simulink model "P1sim"  (R2020b)
settings: Solver=VariableStepAuto  StartTime=0.0  StopTime=100  RelTol=1e-3
undefined symbols (not defined in the file): A, B, C, den, ftDisc, ftPIDdisc, kd1, Kesc, ki, ki2, kp, Kram, num, rampCER, rampPOL, wMuestr
settings Model: Creator=Julian  LastModifiedBy=Julian

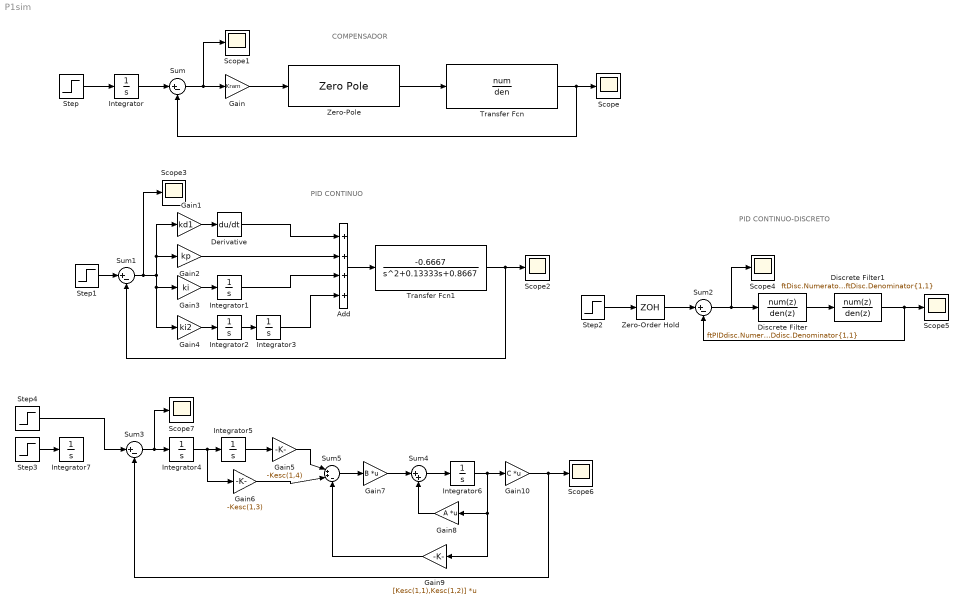
== system P1sim ==
  note: PID CONTINUO-DISCRETO
  note: PID CONTINUO
  note: COMPENSADOR
  Add : Sum  Inputs=++++
  Derivative : Derivative
  Discrete Filter : DiscreteFilter  Numerator=ftPIDdisc.Numerator{1,1}  Denominator=ftPIDdisc.Denominator{1,1}
  Discrete Filter1 : DiscreteFilter  Numerator=ftDisc.Numerator{1,1}  Denominator=ftDisc.Denominator{1,1}
  Gain : Gain  Gain=Kram
  Gain1 : Gain  Gain=kd1
  Gain10 : Gain  Gain=C  Multiplication=Matrix(K*u)
  Gain2 : Gain  Gain=kp
  Gain3 : Gain  Gain=ki
  Gain4 : Gain  Gain=ki2
  Gain5 : Gain  Gain=-Kesc(1,4)
  Gain6 : Gain  Gain=-Kesc(1,3)
  Gain7 : Gain  Gain=B  Multiplication=Matrix(K*u)
  Gain8 : Gain  Gain=A  Multiplication=Matrix(K*u)
  Gain9 : Gain  Gain=[Kesc(1,1),Kesc(1,2)]  Multiplication=Matrix(K*u)
  Integrator{,1..7} (8 alike) : Integrator
  Scope{,1..7} (8 alike) : Scope
  Step : Step  SampleTime=0
  Step{1..4} (4 alike) : Step  Time=0  SampleTime=0
  Sum{,1..3} (4 alike) : Sum  Inputs=|+-
  Sum4 : Sum  Inputs=|++
  Sum5 : Sum  Inputs=|++-
  Transfer Fcn : TransferFcn  Numerator=num  Denominator=den
  Transfer Fcn1 : TransferFcn  Numerator=-0.6667  Denominator=[1 0.13333 0.8667]
  Zero-Order Hold : ZeroOrderHold  SampleTime=wMuestr
  Zero-Pole : ZeroPole  Zeros=rampCER  Poles=rampPOL
  wires:
  Zero-Pole/1 -> Transfer Fcn/1
  Transfer Fcn/1 -> Scope/1, Sum/2
  Sum/1 -> Scope1/1, Gain/1
  Gain/1 -> Zero-Pole/1
  Integrator/1 -> Sum/1
  Step/1 -> Integrator/1
  Gain1/1 -> Derivative/1
  Gain3/1 -> Integrator1/1
  Gain4/1 -> Integrator2/1
  Integrator2/1 -> Integrator3/1
  Add/1 -> Transfer Fcn1/1
  Derivative/1 -> Add/1
  Gain2/1 -> Add/2
  Integrator1/1 -> Add/3
  Integrator3/1 -> Add/4
  Sum1/1 -> Scope3/1, Gain4/1, Gain3/1, Gain1/1, Gain2/1
  Transfer Fcn1/1 -> Scope2/1, Sum1/2
  Step1/1 -> Sum1/1
  Zero-Order Hold/1 -> Sum2/1
  Sum2/1 -> Discrete Filter/1, Scope4/1
  Discrete Filter1/1 -> Scope5/1, Sum2/2
  Discrete Filter/1 -> Discrete Filter1/1
  Step2/1 -> Zero-Order Hold/1
  Sum3/1 -> Scope7/1, Integrator4/1
  Integrator4/1 -> Gain6/1, Integrator5/1
  Integrator5/1 -> Gain5/1
  Gain7/1 -> Sum4/1
  Sum4/1 -> Integrator6/1
  Integrator6/1 -> Gain9/1, Gain8/1, Gain10/1
  Gain8/1 -> Sum4/2
  Gain10/1 -> Scope6/1, Sum3/2
  Step3/1 -> Integrator7/1
  Step4/1 -> Sum3/1
  Gain9/1 -> Sum5/3
  Gain6/1 -> Sum5/2
  Gain5/1 -> Sum5/1
  Sum5/1 -> Gain7/1
